simulink model "ShipCoureControlModel"  (R2020b)
settings: Solver=VariableStepAuto  StartTime=0.0  StopTime=10  RelTol=1e-3
values from neighbouring files (symbols this model uses):
  b0 = -3.42    [InitializeShipModelParameters.m]
  b1 = -7.32    [InitializeShipModelParameters.m]
  b2 = 2.87    [InitializeShipModelParameters.m]
  b3 = 9.77    [InitializeShipModelParameters.m]
  D = 0    [InitializeShipModelParameters.m]    (also in PSO.m = Kd_BEST; RunningModelDemo.m = 0.0001)
  deltaMax = 35    [InitializeShipModelParameters.m]
  I = 0.3    [InitializeShipModelParameters.m]    (also in PSO.m = Ki_BEST; RunningModelDemo.m = 0.001)
  K = 0.061    [InitializeShipModelParameters.m]
  N = 12    [InitializeShipModelParameters.m]
  P = 100    [InitializeShipModelParameters.m]    (also in PSO.m = Kp_BEST; RunningModelDemo.m = 1)
  PB = 5    [InitializeShipModelParameters.m]
  T1 = 83.5    [InitializeShipModelParameters.m]
  T2 = 966.3    [InitializeShipModelParameters.m]
  T3 = 543    [InitializeShipModelParameters.m]
libraries: pid_lib x1
settings Model: Creator=jaqbk  LastModifiedBy=jaqbk

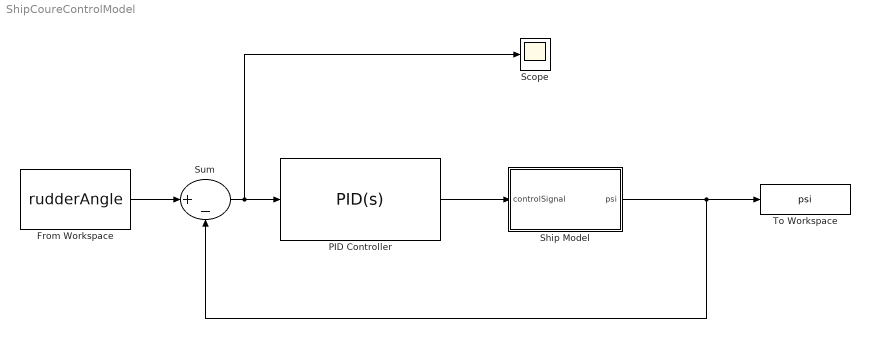
== system ShipCoureControlModel ==
  From Workspace : FromWorkspace  VariableName=rudderAngle  OutputAfterFinalValue=Holding final value
  PID Controller : pid_lib/PID Controller  Controller=PID  Form=Parallel  TimeDomain=Continuous-time  UseExternalTs=off  SampleTime=-1  IntegratorMethod=Forward Euler  FilterMethod=Forward Euler  ControllerParametersSource=internal  P=P  I=I  D=D  UseFilter=on  N=100  TunerSelectOption=Transfer Function Based (PID Tuner App)  InitialConditionSource=internal  InitialConditionForIntegrator=0  InitialConditionForFilter=0  DifferentiatorICPrevScaledInput=0  ExternalReset=none  TrackingMode=off  Kt=1  LimitOutput=off  SatLimitsSource=internal  UpperSaturationLimit=inf  LowerSaturationLimit=-inf  LinearizeAsGain=on  AntiWindupMode=none  Kb=1  POutMin=[]  POutMax=[]  IOutMin=[]  IOutMax=[]  DOutMin=[]  DOutMax=[]  NOutMin=[]  NOutMax=[]  SumOutMin=[]  SumOutMax=[]  SaturationOutMin=[]  SaturationOutMax=[]  PParamMin=[]  PParamMax=[]  IParamMin=[]  IParamMax=[]  DParamMin=[]  DParamMax=[]  NParamMin=[]  NParamMax=[]  KbParamMin=[]  KbParamMax=[]  KtParamMin=[]  KtParamMax=[]  KbOutMin=[]  KbOutMax=[]  KtOutMin=[]  KtOutMax=[]  IntegratorOutMin=[]  IntegratorOutMax=[]  FilterOutMin=[]  FilterOutMax=[]  SumI1OutMin=[]  SumI1OutMax=[]  SumI2OutMin=[]  SumI2OutMax=[]  SumI3OutMin=[]  SumI3OutMax=[]  SumI4OutMin=[]  SumI4OutMax=[]  SumDOutMin=[]  SumDOutMax=[]  DifferentiatorOutMin=[]  DifferentiatorOutMax=[]  FilterDiffOutCoefMin=[]  FilterDiffOutCoefMax=[]  ReciprocalOutMin=[]  ReciprocalOutMax=[]  SumDenOutMin=[]  SumDenOutMax=[]  SumNumOutMin=[]  SumNumOutMax=[]  DivideOutMin=[]  DivideOutMax=[]  UdiffTsProdOutMin=[]  UdiffTsProdOutMax=[]  NTsProdOutMin=[]  NTsProdOutMax=[]  UintegralTsProdOutMin=[]  UintegralTsProdOutMax=[]  UngainTsProdOutMin=[]  UngainTsProdOutMax=[]  IntegratorContinuousStateAttributes=''  IntegratorStateMustResolveToSignalObject=off  IntegratorRTWStateStorageClass=Auto  FilterContinuousStateAttributes=''  FilterStateMustResolveToSignalObject=off  FilterRTWStateStorageClass=Auto  ParallelPVariant=InternalParameters  IdealPVariant=Disabled  IVariant=InternalParameters  DVariant=InternalParameters  IntegratorVariant=Continuous  SatVariant=Disabled  AWVariant=Passthrough  PCopyVariant=Disabled  TRVariant=Disabled  FdbkBlocksVariant=Forward  IdealPFdbkVariant=Disabled  SatFdbkVariant=Disabled  DerivativeFilterVariant=ContFilter  NVariant=InternalParameters  NCopyVariant=Disabled  FilterICVariant=InternalICsFilter  IntegratorICVariant=InternalICs  ExternalResetVariant=Disabled  TRSumVariant=Passthrough  SumFdbkVariant=Disabled  SumVariant=Sum_PID  TsampFilterVariant=InternalTs  TsampNgainVariant=Passthrough  TsampIntegralVariant=Passthrough  ExternalSaturationOutDataTypeStr=Inherit: Same as second input
  Scope : Scope
  Ship Model : Subsystem
  Sum : Sum  Inputs=|+-
  To Workspace : ToWorkspace  VariableName=psi  SampleTime=-1
      settings: Save2DSignal=2-D array (concatenate along first dimension)
  wires:
  Ship Model/1(psi) -> Sum/2, To Workspace/1
  PID Controller/1 -> Ship Model/1(controlSignal)
  Sum/1 -> Scope/1, PID Controller/1
  From Workspace/1 -> Sum/1

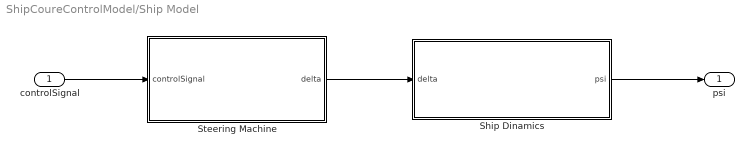
== system ShipCoureControlModel/Ship Model ==
  controlSignal : Inport
  Ship Dinamics : Subsystem
  Steering Machine : Subsystem
  psi : Outport
  wires:
  Steering Machine/1(delta) -> Ship Dinamics/1(delta)
  controlSignal/1 -> Steering Machine/1(controlSignal)
  Ship Dinamics/1(psi) -> psi/1

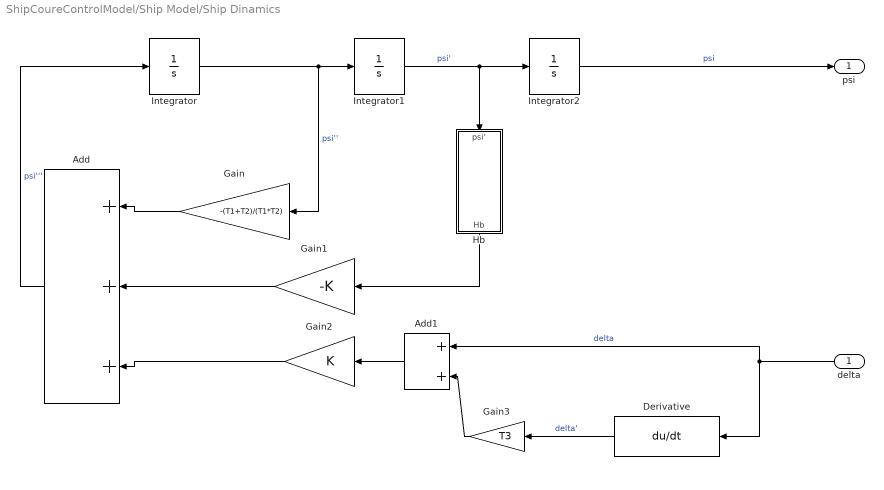
== system ShipCoureControlModel/Ship Model/Ship Dinamics ==
  delta : Inport
  Add : Sum  Inputs=+++
  Add1 : Sum
  Derivative : Derivative
  Gain : Gain  Gain=-(T1+T2)/(T1*T2)
  Gain1 : Gain  Gain=-K
  Gain2 : Gain  Gain=K
  Gain3 : Gain  Gain=T3
  Hb : Subsystem
  Integrator : Integrator
  Integrator1 : Integrator
  Integrator2 : Integrator
  psi : Outport
  wires:
  Gain/1 -> Add/1
  Hb/1(Hb) -> Gain1/1
  Integrator1/1 -> Hb/1(psi'), Integrator2/1  "psi'"
  Integrator2/1 -> psi/1  "psi"
  Integrator/1 -> Gain/1, Integrator1/1  "psi''"
  Gain1/1 -> Add/2
  Add/1 -> Integrator/1  "psi'''"
  Gain2/1 -> Add/3
  delta/1 -> Add1/1, Derivative/1  "delta"
  Derivative/1 -> Gain3/1  "delta'"
  Add1/1 -> Gain2/1
  Gain3/1 -> Add1/2

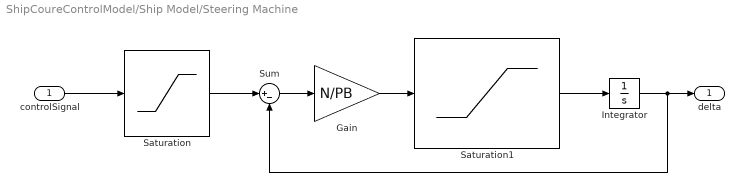
== system ShipCoureControlModel/Ship Model/Steering Machine ==
  controlSignal : Inport
  Gain : Gain  Gain=N/PB
  Integrator : Integrator
  Saturation : Saturate  UpperLimit=deltaMax  LowerLimit=-deltaMax
  Saturation1 : Saturate  UpperLimit=N  LowerLimit=-N
  Sum : Sum  Inputs=|+-
  delta : Outport
  wires:
  controlSignal/1 -> Saturation/1
  Saturation/1 -> Sum/1
  Saturation1/1 -> Integrator/1
  Sum/1 -> Gain/1
  Gain/1 -> Saturation1/1
  Integrator/1 -> Sum/2, delta/1

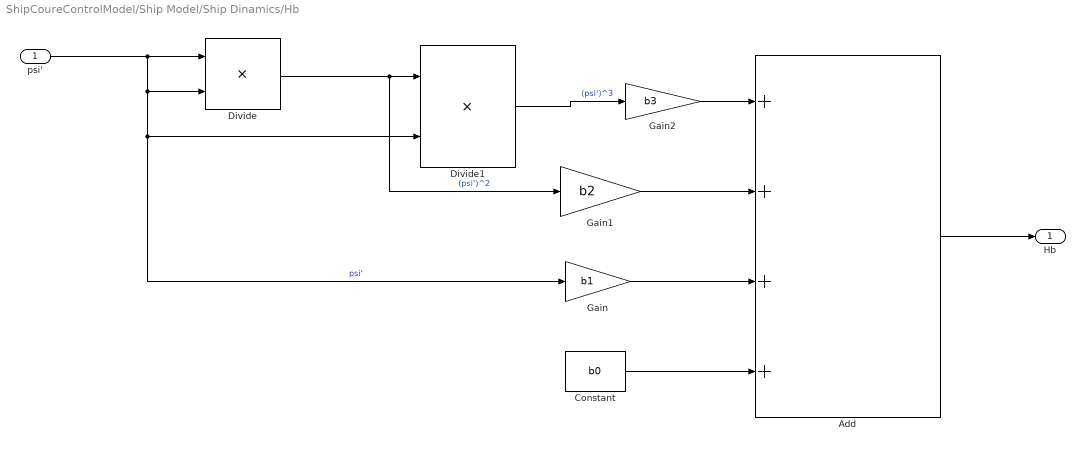
== system ShipCoureControlModel/Ship Model/Ship Dinamics/Hb ==
  psi' : Inport
  Add : Sum  Inputs=++++
  Constant : Constant  Value=b0
  Divide : Product  Inputs=**
  Divide1 : Product  Inputs=**
  Gain : Gain  Gain=b1
  Gain1 : Gain  Gain=b2
  Gain2 : Gain  Gain=b3
  Hb : Outport
  wires:
  psi'/1 -> Gain/1, Divide1/2, Divide/2, Divide/1  "psi'"
  Divide/1 -> Gain1/1, Divide1/1  "(psi')^2"
  Divide1/1 -> Gain2/1  "(psi')^3"
  Constant/1 -> Add/4
  Gain/1 -> Add/3
  Gain2/1 -> Add/1
  Add/1 -> Hb/1
  Gain1/1 -> Add/2
